simulink model "fuzzytfg"  (R2020b)
settings: Solver=VariableStepAuto  StartTime=0.0  StopTime=20.0  RelTol=1e-3
libraries: fuzblock x1
settings Model: Creator=diosdado  LastModifiedBy=diosdado

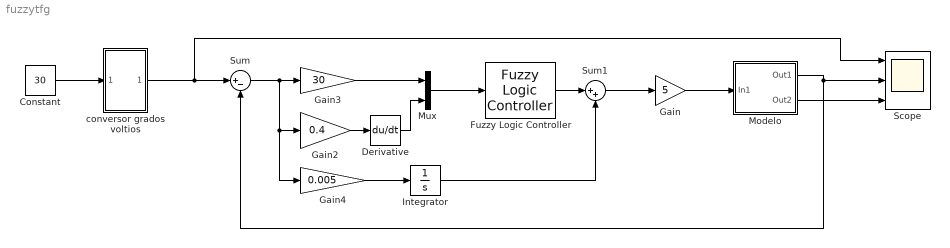
== system fuzzytfg ==
  Constant : Constant  Value=30
  Derivative : Derivative
  Fuzzy Logic Controller : fuzblock/Fuzzy Logic  Controller  FIS='FUZZY3.fis'  OutputSampleNumber=101  DataType=double  FuzzifiedInputs=off  RuleFiringStrengths=off  RuleOutputs=off  AggregatedOutputs=off  SimulateUsing=Interpreted execution  OutOfRangeInputValueMessage=warning  NoRuleFiredMessage=warning  EmptyOutputFuzzySetMessage=warning
  Gain : Gain  Gain=5
  Gain2 : Gain  Gain=0.4
  Gain3 : Gain  Gain=30
  Gain4 : Gain  Gain=0.005
  Integrator : Integrator
  "Modelo " : Subsystem
  Mux : Mux  Inputs=2
  Scope : Scope  NumInputPorts=3
  Sum : Sum  Inputs=|+-
  Sum1 : Sum  Inputs=|++
  "conversor grados voltios " : Subsystem  mask{a=4.95, b=0.869}
  wires:
  Constant/1 -> "conversor grados voltios "/1(In1)
  Sum/1 -> Gain3/1, Gain2/1, Gain4/1
  Mux/1 -> Fuzzy Logic Controller/1
  Derivative/1 -> Mux/2
  Gain/1 -> "Modelo "/1(In1)
  "Modelo "/1(Out1) -> Sum/2, Scope/2
  "Modelo "/2(Out2) -> Scope/3
  "conversor grados voltios "/1(Out1) -> Scope/1, Sum/1
  Gain3/1 -> Mux/1
  Fuzzy Logic Controller/1 -> Sum1/1
  Sum1/1 -> Gain/1
  Integrator/1 -> Sum1/2
  Gain4/1 -> Integrator/1
  Gain2/1 -> Derivative/1

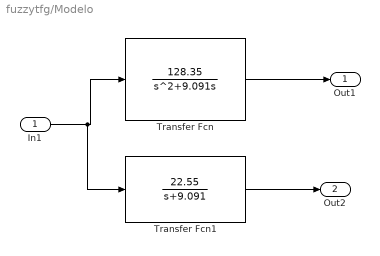
== system fuzzytfg/Modelo  ==
  In1 : Inport
  Transfer Fcn : TransferFcn  Numerator=[128.35]  Denominator=[1 9.091 0]
  Transfer Fcn1 : TransferFcn  Numerator=[22.55]  Denominator=[1 9.091]
  Out1 : Outport
  Out2 : Outport  Port=2
  wires:
  In1/1 -> Transfer Fcn1/1, Transfer Fcn/1
  Transfer Fcn/1 -> Out1/1
  Transfer Fcn1/1 -> Out2/1

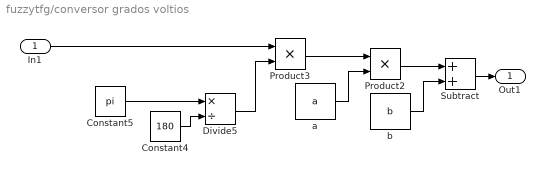
== system fuzzytfg/conversor grados voltios  ==
  In1 : Inport
  Constant4 : Constant  Value=180
  Constant5 : Constant  Value=pi
  Divide5 : Product  Inputs=*/
  Product2 : Product
  Product3 : Product
  Subtract : Sum
  a : Constant  Value=a
  b : Constant  Value=b
  Out1 : Outport
  wires:
  b/1 -> Subtract/2
  Product3/1 -> Product2/1
  Constant4/1 -> Divide5/2
  In1/1 -> Product3/1
  Product2/1 -> Subtract/1
  a/1 -> Product2/2
  Constant5/1 -> Divide5/1
  Divide5/1 -> Product3/2
  Subtract/1 -> Out1/1
